simulink model "fast_test_linAnalisis"  (R2017a)
settings: Solver=VariableStepAuto  StartTime=0.0  StopTime=.2  MaxStep=1e-6  RelTol=1e-3
undefined symbols (not defined in the file or in its folder): hx
libraries: simulink_extras x2
settings Model: Creator=erich  LastModifiedBy=erich

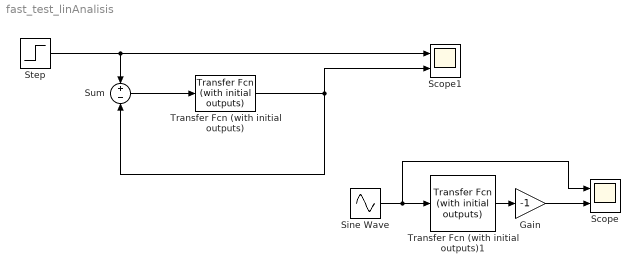
== system fast_test_linAnalisis ==
  Gain : Gain  Gain=-1
  Scope : Scope  NumInputPorts=2
  Scope1 : Scope  NumInputPorts=2
  Sine Wave : Sin  Amplitude=10  Frequency=2*pi*60  SampleTime=0
  Step : Step  Time=0  SampleTime=0
  Sum : Sum  Inputs=+-
  Transfer Fcn (with initial outputs) : simulink_extras/Additional Linear/Transfer Fcn (with initial outputs)  N=[1]  D="[1  1]"  Y0=0  U0=0
  Transfer Fcn (with initial outputs)1 : simulink_extras/Additional Linear/Transfer Fcn (with initial outputs)  N=cell2mat(hx.Numerator)  D=cell2mat(hx.Denominator)  Y0=0  U0=0
  wires:
  Sum/1 -> Transfer Fcn (with initial outputs)/1
  Transfer Fcn (with initial outputs)/1 -> Sum/2, Scope1/2
  Step/1 -> Sum/1, Scope1/1
  Sine Wave/1 -> Scope/1, Transfer Fcn (with initial outputs)1/1
  Transfer Fcn (with initial outputs)1/1 -> Gain/1
  Gain/1 -> Scope/2
